simulink model "Torque_regulation_1_1"  (R2022b)
settings: Solver=FixedStepAuto  StartTime=0.0  StopTime=10  FixedStep=0.01  RelTol=1e-3
libraries: simulink x6, dspstat3 x4, eeGeneralControl x4, slpidlib x2
settings Model: Creator=tiszu  LastModifiedBy=tiszu

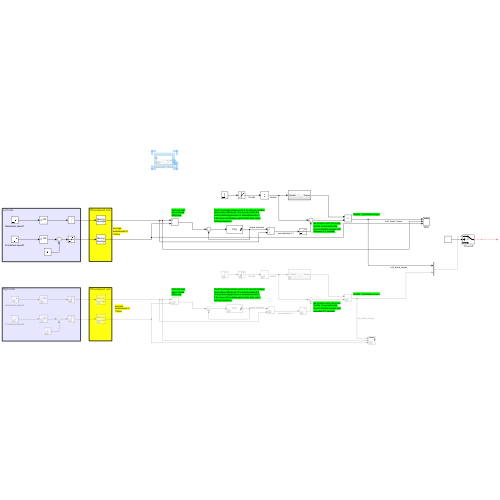
[thumbnail: Simulink's stored preview of the top-level diagram]
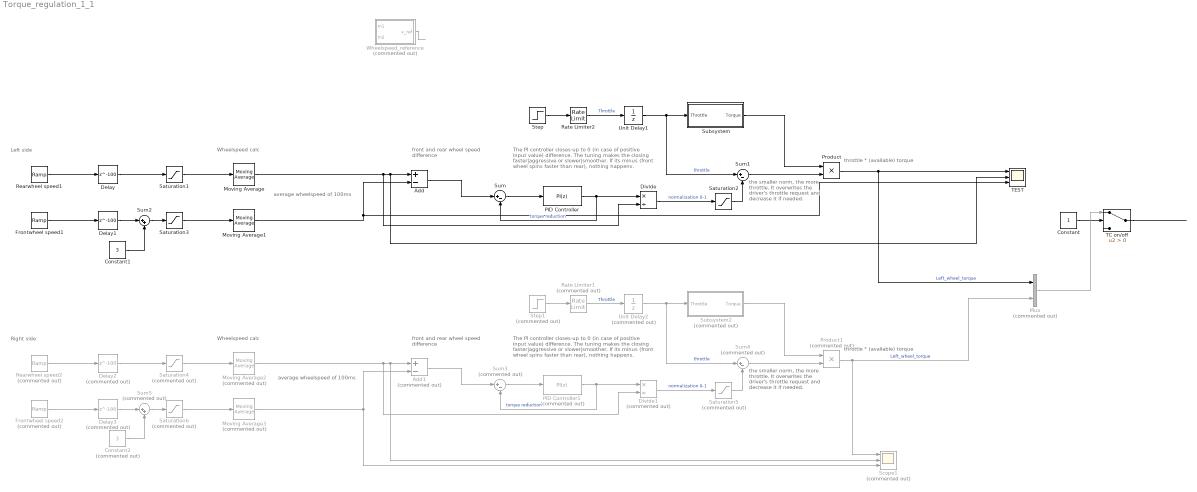
== system Torque_regulation_1_1 ==
  note: throttle * (available) torque
  note: the smaller norm, the more throttle. It overwrites the driver's throttle request and decrease it if needed.
  note: The PI controller closes-up to 0 (in case of positive input value) difference. The tuning makes the closing faster|aggressive or slower|smoother.
      | If its minus (front wheel spins faster than rear), nothing happens.
  note: average wheelspeed of 100ms
  note: Wheelspeed calc
  note: front and rear wheel speed difference
  note: Left side
  note: the smaller norm, the more throttle. It overwrites the driver's throttle request and decrease it if needed.
  note: Right side
  note: average wheelspeed of 100ms
  note: throttle * (available) torque
  note: The PI controller closes-up to 0 (in case of positive input value) difference. The tuning makes the closing faster|aggressive or slower|smoother.
      | If its minus (front wheel spins faster than rear), nothing happens.
  note: Wheelspeed calc
  note: front and rear wheel speed difference
  Add : Sum  Inputs=+-
  Add1 : Sum  Commented=on  Inputs=+-
  Constant : Constant
  Constant1 : Constant  Value=3
  Constant2 : Constant  Commented=on  Value=3
  Delay : Delay  DelayLength=100
  Delay1 : Delay  DelayLength=100
  Delay2 : Delay  Commented=on  DelayLength=100
  Delay3 : Delay  Commented=on  DelayLength=100
  Divide : Product  Inputs=*/
  Divide1 : Product  Commented=on  Inputs=*/
  Frontwheel speed1 : simulink/Sources/Ramp  slope=10  start=0  InitialOutput=0
  Frontwheel speed2 : simulink/Sources/Ramp  Commented=on  slope=10  start=0  InitialOutput=0
  Moving Average : dspstat3/Moving Average  Method=Sliding window  ForgettingFactorPort=off  SpecifyWindowLength=on  WindowLength=100  OverlapLength=99  AllowArbitraryInputLength=off  ForgettingFactor=0.9  SimulateUsing=Code generation
  Moving Average1 : dspstat3/Moving Average  Method=Sliding window  ForgettingFactorPort=off  SpecifyWindowLength=on  WindowLength=100  OverlapLength=99  AllowArbitraryInputLength=off  ForgettingFactor=0.9  SimulateUsing=Code generation
  Moving Average2 : dspstat3/Moving Average  Commented=on  Method=Sliding window  ForgettingFactorPort=off  SpecifyWindowLength=on  WindowLength=100  OverlapLength=99  AllowArbitraryInputLength=off  ForgettingFactor=0.9  SimulateUsing=Code generation
  Moving Average3 : dspstat3/Moving Average  Commented=on  Method=Sliding window  ForgettingFactorPort=off  SpecifyWindowLength=on  WindowLength=100  OverlapLength=99  AllowArbitraryInputLength=off  ForgettingFactor=0.9  SimulateUsing=Code generation
  Mux : Mux  Commented=on  Inputs=2
  PID Controller : slpidlib/PID Controller  Controller=PI  Form=Parallel  TimeDomain=Discrete-time  UseExternalTs=off  SampleTime=0.01  IntegratorMethod=Forward Euler  FilterMethod=Forward Euler  ControllerParametersSource=internal  P=1  I=2  UseKiTs=off  D=0  N=100  UseFilter=on  TunerSelectOption=Transfer Function Based (PID Tuner App)  InitialConditionSource=internal  InitialConditionForIntegrator=0  InitialConditionForFilter=0  DifferentiatorICPrevScaledInput=0  ExternalReset=none  TrackingMode=off  Kt=1  LimitOutput=on  SatLimitsSource=internal  UpperSaturationLimit=100  LowerSaturationLimit=0  LinearizeAsGain=on  AntiWindupMode=clamping  Kb=1  LimitIntegrator=off  UpperIntegratorSaturationLimit=inf  LowerIntegratorSaturationLimit=-inf  POutMin=[]  POutMax=[]  IOutMin=[]  IOutMax=[]  DOutMin=[]  DOutMax=[]  NOutMin=[]  NOutMax=[]  SumOutMin=[]  SumOutMax=[]  SaturationOutMin=[]  SaturationOutMax=[]  PParamMin=[]  PParamMax=[]  IParamMin=[]  IParamMax=[]  DParamMin=[]  DParamMax=[]  NParamMin=[]  NParamMax=[]  KbParamMin=[]  KbParamMax=[]  KtParamMin=[]  KtParamMax=[]  KbOutMin=[]  KbOutMax=[]  KtOutMin=[]  KtOutMax=[]  IntegratorOutMin=[]  IntegratorOutMax=[]  FilterOutMin=[]  FilterOutMax=[]  SumI1OutMin=[]  SumI1OutMax=[]  SumI2OutMin=[]  SumI2OutMax=[]  SumI3OutMin=[]  SumI3OutMax=[]  SumI4OutMin=[]  SumI4OutMax=[]  SumDOutMin=[]  SumDOutMax=[]  DifferentiatorOutMin=[]  DifferentiatorOutMax=[]  FilterDiffOutCoefMin=[]  FilterDiffOutCoefMax=[]  ReciprocalOutMin=[]  ReciprocalOutMax=[]  SumDenOutMin=[]  SumDenOutMax=[]  SumNumOutMin=[]  SumNumOutMax=[]  DivideOutMin=[]  DivideOutMax=[]  UdiffTsProdOutMin=[]  UdiffTsProdOutMax=[]  NTsProdOutMin=[]  NTsProdOutMax=[]  UintegralTsProdOutMin=[]  UintegralTsProdOutMax=[]  UngainTsProdOutMin=[]  UngainTsProdOutMax=[]  ClampingZeroOutDataTypeStr=Inherit: Inherit via back propagation  ClampingZeroOutMin=[]  ClampingZeroOutMax=[]  FilterDenConstantOutDataTypeStr=Inherit: Inherit via back propagation  FilterDenConstantOutMin=[]  FilterDenConstantOutMax=[]  PCopyOutDataTypeStr=Inherit: Inherit via back propagation  PCopyOutMin=[]  PCopyOutMax=[]  NCopyOutDataTypeStr=Inherit: Inherit via back propagation  NCopyOutMin=[]  NCopyOutMax=[]  IntegratorContinuousStateAttributes=''  IntegratorStateMustResolveToSignalObject=off  IntegratorRTWStateStorageClass=Auto  FilterContinuousStateAttributes=''  FilterStateMustResolveToSignalObject=off  FilterRTWStateStorageClass=Auto  ParallelPVariant=InternalParameters  IdealPVariant=Disabled  IVariant=InternalParameters  DVariant=Disabled  IntegratorVariant=Discrete  SatVariant=Enabled  AWVariant=DiscClampingParallel  PCopyVariant=Disabled  TRVariant=Disabled  FdbkBlocksVariant=Forward  IdealPFdbkVariant=Disabled  SatFdbkVariant=Disabled  DerivativeFilterVariant=Disabled  NVariant=Disabled  NCopyVariant=Disabled_SignalSpec  FilterICVariant=Disabled  IntegratorICVariant=InternalICs  ExternalResetVariant=Disabled  TRSumVariant=Passthrough  SumFdbkVariant=Disabled  SumVariant=Sum_PI  TsampFilterVariant=InternalTs  TsampNgainVariant=Passthrough  TsampIntegralVariant=Passthrough  ExternalSaturationOutDataTypeStr=Inherit: Same as second input
  PID Controller1 : slpidlib/PID Controller  Commented=on  Controller=PI  Form=Parallel  TimeDomain=Discrete-time  UseExternalTs=off  SampleTime=0.01  IntegratorMethod=Forward Euler  FilterMethod=Forward Euler  ControllerParametersSource=internal  P=1  I=2  UseKiTs=off  D=0  N=100  UseFilter=on  TunerSelectOption=Transfer Function Based (PID Tuner App)  InitialConditionSource=internal  InitialConditionForIntegrator=0  InitialConditionForFilter=0  DifferentiatorICPrevScaledInput=0  ExternalReset=none  TrackingMode=off  Kt=1  LimitOutput=on  SatLimitsSource=internal  UpperSaturationLimit=100  LowerSaturationLimit=0  LinearizeAsGain=on  AntiWindupMode=clamping  Kb=1  LimitIntegrator=off  UpperIntegratorSaturationLimit=inf  LowerIntegratorSaturationLimit=-inf  POutMin=[]  POutMax=[]  IOutMin=[]  IOutMax=[]  DOutMin=[]  DOutMax=[]  NOutMin=[]  NOutMax=[]  SumOutMin=[]  SumOutMax=[]  SaturationOutMin=[]  SaturationOutMax=[]  PParamMin=[]  PParamMax=[]  IParamMin=[]  IParamMax=[]  DParamMin=[]  DParamMax=[]  NParamMin=[]  NParamMax=[]  KbParamMin=[]  KbParamMax=[]  KtParamMin=[]  KtParamMax=[]  KbOutMin=[]  KbOutMax=[]  KtOutMin=[]  KtOutMax=[]  IntegratorOutMin=[]  IntegratorOutMax=[]  FilterOutMin=[]  FilterOutMax=[]  SumI1OutMin=[]  SumI1OutMax=[]  SumI2OutMin=[]  SumI2OutMax=[]  SumI3OutMin=[]  SumI3OutMax=[]  SumI4OutMin=[]  SumI4OutMax=[]  SumDOutMin=[]  SumDOutMax=[]  DifferentiatorOutMin=[]  DifferentiatorOutMax=[]  FilterDiffOutCoefMin=[]  FilterDiffOutCoefMax=[]  ReciprocalOutMin=[]  ReciprocalOutMax=[]  SumDenOutMin=[]  SumDenOutMax=[]  SumNumOutMin=[]  SumNumOutMax=[]  DivideOutMin=[]  DivideOutMax=[]  UdiffTsProdOutMin=[]  UdiffTsProdOutMax=[]  NTsProdOutMin=[]  NTsProdOutMax=[]  UintegralTsProdOutMin=[]  UintegralTsProdOutMax=[]  UngainTsProdOutMin=[]  UngainTsProdOutMax=[]  ClampingZeroOutDataTypeStr=Inherit: Inherit via back propagation  ClampingZeroOutMin=[]  ClampingZeroOutMax=[]  FilterDenConstantOutDataTypeStr=Inherit: Inherit via back propagation  FilterDenConstantOutMin=[]  FilterDenConstantOutMax=[]  PCopyOutDataTypeStr=Inherit: Inherit via back propagation  PCopyOutMin=[]  PCopyOutMax=[]  NCopyOutDataTypeStr=Inherit: Inherit via back propagation  NCopyOutMin=[]  NCopyOutMax=[]  IntegratorContinuousStateAttributes=''  IntegratorStateMustResolveToSignalObject=off  IntegratorRTWStateStorageClass=Auto  FilterContinuousStateAttributes=''  FilterStateMustResolveToSignalObject=off  FilterRTWStateStorageClass=Auto  ParallelPVariant=InternalParameters  IdealPVariant=Disabled  IVariant=InternalParameters  DVariant=Disabled  IntegratorVariant=Discrete  SatVariant=Enabled  AWVariant=DiscClampingParallel  PCopyVariant=Disabled  TRVariant=Disabled  FdbkBlocksVariant=Forward  IdealPFdbkVariant=Disabled  SatFdbkVariant=Disabled  DerivativeFilterVariant=Disabled  NVariant=Disabled  NCopyVariant=Disabled_SignalSpec  FilterICVariant=Disabled  IntegratorICVariant=InternalICs  ExternalResetVariant=Disabled  TRSumVariant=Passthrough  SumFdbkVariant=Disabled  SumVariant=Sum_PI  TsampFilterVariant=InternalTs  TsampNgainVariant=Passthrough  TsampIntegralVariant=Passthrough  ExternalSaturationOutDataTypeStr=Inherit: Same as second input
  Product : Product
  Product1 : Product  Commented=on
  Rate Limiter1 : RateLimiter  Commented=on  SampleTimeMode=inherited
  Rate Limiter2 : RateLimiter  SampleTimeMode=inherited
  Rearwheel speed1 : simulink/Sources/Ramp  slope=50  start=0  InitialOutput=0
  Rearwheel speed2 : simulink/Sources/Ramp  Commented=on  slope=50  start=0  InitialOutput=0
  Saturation1 : Saturate  UpperLimit=30  LowerLimit=0
  Saturation2 : Saturate  UpperLimit=1  LowerLimit=0
  Saturation3 : Saturate  UpperLimit=30  LowerLimit=0
  Saturation4 : Saturate  Commented=on  UpperLimit=30  LowerLimit=0
  Saturation5 : Saturate  Commented=on  UpperLimit=1  LowerLimit=0
  Saturation6 : Saturate  Commented=on  UpperLimit=30  LowerLimit=0
  Scope1 : Scope  Commented=on  NumInputPorts=3
  Step : Step  SampleTime=0
  Step1 : Step  Commented=on  SampleTime=0
  Subsystem : Subsystem
  Subsystem2 : Subsystem  Commented=on
  Sum : Sum  Inputs=|+-
  Sum1 : Sum  Inputs=|+-
  Sum2 : Sum  Inputs=|++
  Sum3 : Sum  Commented=on  Inputs=|+-
  Sum4 : Sum  Commented=on  Inputs=|+-
  Sum5 : Sum  Commented=on  Inputs=|++
  TC on/off : Switch  Criteria=u2 > Threshold  SaturateOnIntegerOverflow=off  InputSameDT=off
  TEST : Scope  NumInputPorts=3
  Unit Delay1 : UnitDelay  SampleTime=-1  HasFrameUpgradeWarning=on
  Unit Delay2 : UnitDelay  Commented=on  SampleTime=-1  HasFrameUpgradeWarning=on
  Wheelspeed_reference : Subsystem  Commented=on
  wires:
  Subsystem/1(Torque) -> Product/1
  Divide/1 -> Saturation2/1  "normalization 0-1"
  Sum1/1 -> Product/2
  PID Controller/1 -> Sum/2, Divide/1  "torque reduction"
  Saturation2/1 -> Sum1/2
  Wheelspeed_reference/1(v_ref) -> ?
  Sum2/1 -> Saturation3/1
  Sum/1 -> PID Controller/1
  Add/1 -> Sum/1
  Saturation1/1 -> Moving Average/1
  Saturation3/1 -> Moving Average1/1
  Delay/1 -> Saturation1/1
  Delay1/1 -> Sum2/1
  Rearwheel speed1/1 -> Delay/1
  Frontwheel speed1/1 -> Delay1/1
  Step/1 -> Rate Limiter2/1
  Rate Limiter2/1 -> Unit Delay1/1  "Throttle"
  Unit Delay1/1 -> Sum1/1, Subsystem/1(Throttle)  "throttle"
  Constant/1 -> TC on/off/2
  Mux/1 -> TC on/off/1
  TC on/off/1 -> ?
  Product/1 -> TEST/1, Mux/1  "Left_wheel_torque"
  Constant1/1 -> Sum2/2
  Moving Average/1 -> Divide/2, TEST/2, Add/1
  Moving Average1/1 -> Add/2, TEST/3
  Frontwheel speed2/1 -> Delay3/1
  Rate Limiter1/1 -> Unit Delay2/1  "Throttle"
  Subsystem2/1(Torque) -> Product1/1
  Sum4/1 -> Product1/2
  Unit Delay2/1 -> Sum4/1, Subsystem2/1(Throttle)  "throttle"
  Product1/1 -> Scope1/1, Mux/2  "Left_wheel_torque"
  Moving Average3/1 -> Add1/2, Scope1/3
  Constant2/1 -> Sum5/2
  Rearwheel speed2/1 -> Delay2/1
  Moving Average2/1 -> Divide1/2, Scope1/2, Add1/1
  Step1/1 -> Rate Limiter1/1
  Saturation6/1 -> Moving Average3/1
  Delay3/1 -> Sum5/1
  Delay2/1 -> Saturation4/1
  Saturation5/1 -> Sum4/2
  Sum3/1 -> PID Controller1/1
  Divide1/1 -> Saturation5/1  "normalization 0-1"
  Add1/1 -> Sum3/1
  Saturation4/1 -> Moving Average2/1
  Sum5/1 -> Saturation6/1
  PID Controller1/1 -> Sum3/2, Divide1/1  "torque reduction"

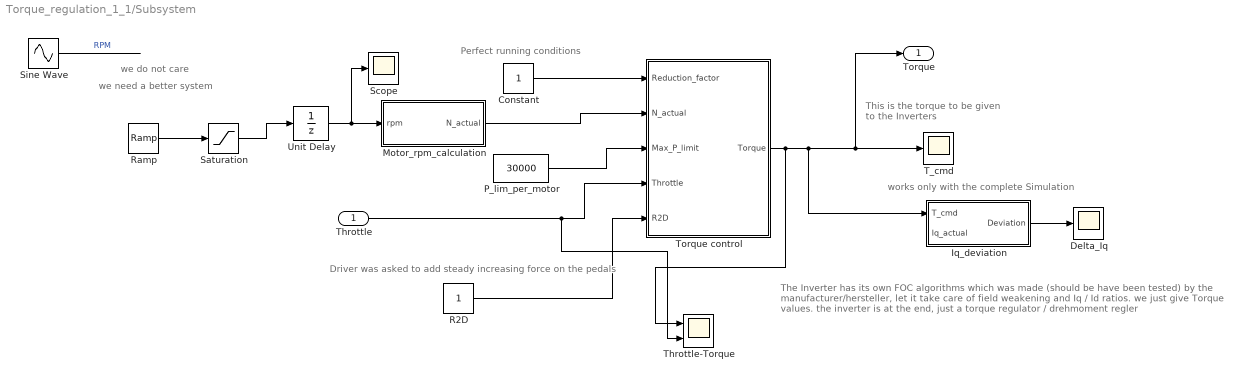
== system Torque_regulation_1_1/Subsystem ==
  note: we need a better system
  note: works only with the complete Simulation
  note: Perfect running conditions
  note: we do not care
  note: Driver was asked to add steady increasing force on the pedals
  note: The Inverter has its own FOC algorithms which was made (should be have been tested) by the manufacturer/hersteller, let it take care of field weakening and Iq / Id ratios. we just give Torque values. the inverter is at the end, just a torque regulator / drehmoment regler
  note: This is the torque to
      | be given to the Inverters
  Throttle : Inport
  Constant : Constant
  Delta_Iq : Scope
  Iq_deviation : Subsystem
  Motor_rpm_calculation : Subsystem
  P_lim_per_motor : Constant  Value=30000
  R2D : Constant
  Ramp : simulink/Sources/Ramp  slope=1000  start=0  InitialOutput=0
  Saturation : Saturate  UpperLimit=2000  LowerLimit=0
  Scope : Scope
  Sine Wave : Sin  Amplitude=2000  SampleTime=0
  T_cmd : Scope
  Throttle-Torque : Scope  NumInputPorts=2
  Torque control : Subsystem
  Unit Delay : UnitDelay  SampleTime=-1  HasFrameUpgradeWarning=on
  Torque : Outport
  wires:
  Throttle/1 -> Throttle-Torque/2, Torque control/4(Throttle)
  R2D/1 -> Torque control/5(R2D)
  Torque control/1(Torque) -> Iq_deviation/1(T_cmd), Torque/1, T_cmd/1, Throttle-Torque/1
  Unit Delay/1 -> Scope/1, Motor_rpm_calculation/1(rpm)
  Iq_deviation/1(Deviation) -> Delta_Iq/1
  Motor_rpm_calculation/1(N_actual) -> Torque control/2(N_actual)
  Sine Wave/1 -> ?  "RPM"
  Ramp/1 -> Saturation/1
  P_lim_per_motor/1 -> Torque control/3(Max_P_limit)
  Saturation/1 -> Unit Delay/1
  Constant/1 -> Torque control/1(Reduction_factor)

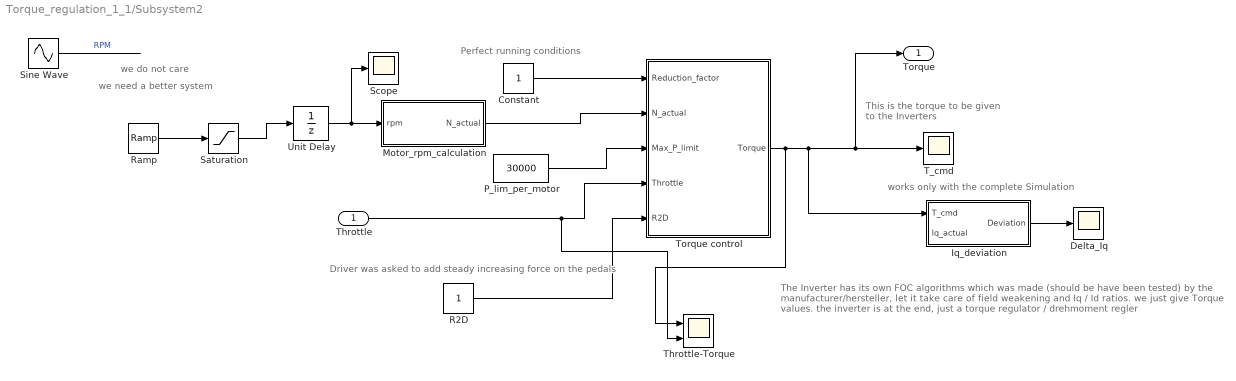
== system Torque_regulation_1_1/Subsystem2 ==
  note: we need a better system
  note: works only with the complete Simulation
  note: Perfect running conditions
  note: we do not care
  note: Driver was asked to add steady increasing force on the pedals
  note: The Inverter has its own FOC algorithms which was made (should be have been tested) by the manufacturer/hersteller, let it take care of field weakening and Iq / Id ratios. we just give Torque values. the inverter is at the end, just a torque regulator / drehmoment regler
  note: This is the torque to
      | be given to the Inverters
  Throttle : Inport
  Constant : Constant
  Delta_Iq : Scope
  Iq_deviation : Subsystem
  Motor_rpm_calculation : Subsystem
  P_lim_per_motor : Constant  Value=30000
  R2D : Constant
  Ramp : simulink/Sources/Ramp  slope=1000  start=0  InitialOutput=0
  Saturation : Saturate  UpperLimit=2000  LowerLimit=0
  Scope : Scope
  Sine Wave : Sin  Amplitude=2000  SampleTime=0
  T_cmd : Scope
  Throttle-Torque : Scope  NumInputPorts=2
  Torque control : Subsystem
  Unit Delay : UnitDelay  SampleTime=-1  HasFrameUpgradeWarning=on
  Torque : Outport
  wires:
  Throttle/1 -> Throttle-Torque/2, Torque control/4(Throttle)
  R2D/1 -> Torque control/5(R2D)
  Torque control/1(Torque) -> Iq_deviation/1(T_cmd), Torque/1, T_cmd/1, Throttle-Torque/1
  Unit Delay/1 -> Scope/1, Motor_rpm_calculation/1(rpm)
  Iq_deviation/1(Deviation) -> Delta_Iq/1
  Motor_rpm_calculation/1(N_actual) -> Torque control/2(N_actual)
  Sine Wave/1 -> ?  "RPM"
  Ramp/1 -> Saturation/1
  P_lim_per_motor/1 -> Torque control/3(Max_P_limit)
  Saturation/1 -> Unit Delay/1
  Constant/1 -> Torque control/1(Reduction_factor)

== system Torque_regulation_1_1/Wheelspeed_reference ==
  In1 : Inport
  In2 : Inport  Port=2
  Min : MinMax  Inputs=2
  v_ref : Outport
  wires:
  In1/1 -> Min/1
  Min/1 -> v_ref/1
  In2/1 -> Min/2

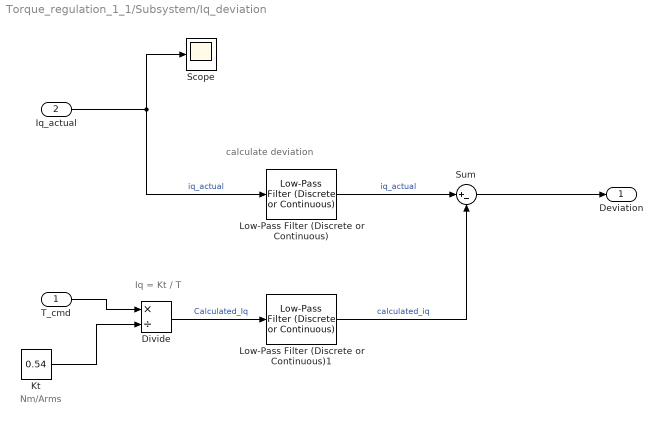
== system Torque_regulation_1_1/Subsystem/Iq_deviation ==
  note: calculate deviation
  note: Iq = Kt / T
  note: Nm/Arms
  T_cmd : Inport
  Iq_actual : Inport  Port=2
  Divide : Product  Inputs=*/
  Kt : Constant  Value=0.54
  Low-Pass Filter (Discrete or Continuous) : eeGeneralControl/Low-Pass Filter (Discrete or Continuous)  K=1  T=1  B=inf  A=-inf  init_option=Inherited from block input  x0=0  Ts=-1
  Low-Pass Filter (Discrete or Continuous)1 : eeGeneralControl/Low-Pass Filter (Discrete or Continuous)  K=1  T=1  B=inf  A=-inf  init_option=Inherited from block input  x0=0  Ts=-1
  Scope : Scope
  Sum : Sum  Inputs=|+-
  Deviation : Outport
  wires:
  Kt/1 -> Divide/2
  T_cmd/1 -> Divide/1
  Iq_actual/1 -> Low-Pass Filter (Discrete or Continuous)/1, Scope/1  "iq_actual"
  Divide/1 -> Low-Pass Filter (Discrete or Continuous)1/1  "Calculated_Iq"
  Sum/1 -> Deviation/1
  Low-Pass Filter (Discrete or Continuous)/1 -> Sum/1  "iq_actual"
  Low-Pass Filter (Discrete or Continuous)1/1 -> Sum/2  "calculated_iq"

== system Torque_regulation_1_1/Subsystem/Motor_rpm_calculation ==
  note: From CAN Docs Pg 19
      | (Unitek)
  rpm : Inport
  15-Bit_Max_value : Constant  Value=32767
  Constant : Constant  Value=8000
  Divide : Product  Inputs=*/
  Product : Product
  N_actual : Outport
  wires:
  rpm/1 -> Divide/1
  Divide/1 -> Product/1
  15-Bit_Max_value/1 -> Product/2
  Constant/1 -> Divide/2
  Product/1 -> N_actual/1

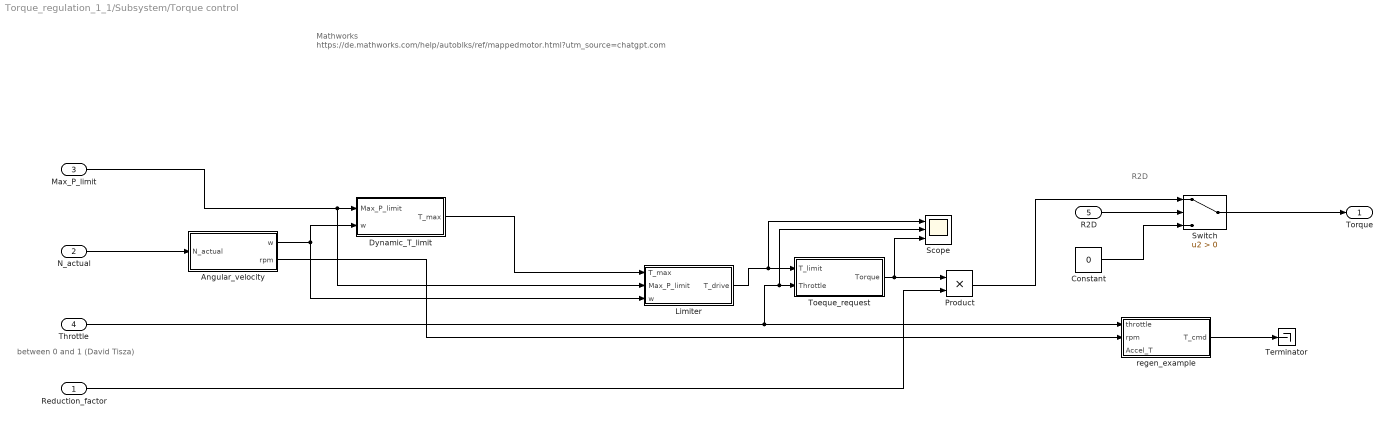
== system Torque_regulation_1_1/Subsystem/Torque control ==
  note: R2D
  note: between 0 and 1 (David Tisza)
  note: Mathworks
      | https://de.mathworks.com/help/autoblks/ref/mappedmotor.html?utm_source=chatgpt.com
  Reduction_factor : Inport
  N_actual : Inport  Port=2
  Max_P_limit : Inport  Port=3
  Throttle : Inport  Port=4
  R2D : Inport  Port=5
  Angular_velocity : Subsystem
  Constant : Constant  Value=0
  Dynamic_T_limit : Subsystem
  Limiter : Subsystem
  Product : Product
  Scope : Scope  NumInputPorts=3
  Switch : Switch  Criteria=u2 > Threshold  SaturateOnIntegerOverflow=off  InputSameDT=off
  Terminator : Terminator
  Toeque_request : Subsystem
  regen_example : Subsystem
  Torque : Outport
  wires:
  N_actual/1 -> Angular_velocity/1(N_actual)
  Throttle/1 -> regen_example/1(throttle), Scope/2, Toeque_request/2(Throttle)
  Angular_velocity/1(w) -> Limiter/3(w), Dynamic_T_limit/2(w)
  Max_P_limit/1 -> Limiter/2(Max_P_limit), Dynamic_T_limit/1(Max_P_limit)
  Limiter/1(T_drive) -> Scope/1, Toeque_request/1(T_limit)
  Toeque_request/1(Torque) -> Scope/3, Product/1
  Product/1 -> Switch/1
  Reduction_factor/1 -> Product/2
  Dynamic_T_limit/1(T_max) -> Limiter/1(T_max)
  Angular_velocity/2(rpm) -> regen_example/2(rpm)
  regen_example/1(T_cmd) -> Terminator/1
  R2D/1 -> Switch/2
  Constant/1 -> Switch/3
  Switch/1 -> Torque/1

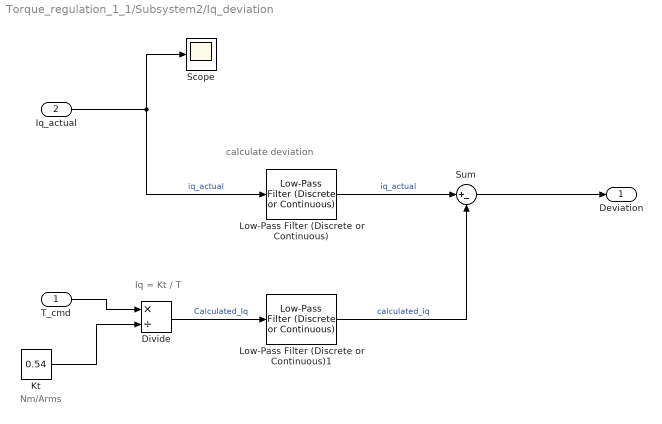
== system Torque_regulation_1_1/Subsystem2/Iq_deviation ==
  note: calculate deviation
  note: Iq = Kt / T
  note: Nm/Arms
  T_cmd : Inport
  Iq_actual : Inport  Port=2
  Divide : Product  Inputs=*/
  Kt : Constant  Value=0.54
  Low-Pass Filter (Discrete or Continuous) : eeGeneralControl/Low-Pass Filter (Discrete or Continuous)  K=1  T=1  B=inf  A=-inf  init_option=Inherited from block input  x0=0  Ts=-1
  Low-Pass Filter (Discrete or Continuous)1 : eeGeneralControl/Low-Pass Filter (Discrete or Continuous)  K=1  T=1  B=inf  A=-inf  init_option=Inherited from block input  x0=0  Ts=-1
  Scope : Scope
  Sum : Sum  Inputs=|+-
  Deviation : Outport
  wires:
  Kt/1 -> Divide/2
  T_cmd/1 -> Divide/1
  Iq_actual/1 -> Low-Pass Filter (Discrete or Continuous)/1, Scope/1  "iq_actual"
  Divide/1 -> Low-Pass Filter (Discrete or Continuous)1/1  "Calculated_Iq"
  Sum/1 -> Deviation/1
  Low-Pass Filter (Discrete or Continuous)/1 -> Sum/1  "iq_actual"
  Low-Pass Filter (Discrete or Continuous)1/1 -> Sum/2  "calculated_iq"

== system Torque_regulation_1_1/Subsystem2/Motor_rpm_calculation ==
  note: From CAN Docs Pg 19
      | (Unitek)
  rpm : Inport
  15-Bit_Max_value : Constant  Value=32767
  Constant : Constant  Value=8000
  Divide : Product  Inputs=*/
  Product : Product
  N_actual : Outport
  wires:
  rpm/1 -> Divide/1
  Divide/1 -> Product/1
  15-Bit_Max_value/1 -> Product/2
  Constant/1 -> Divide/2
  Product/1 -> N_actual/1

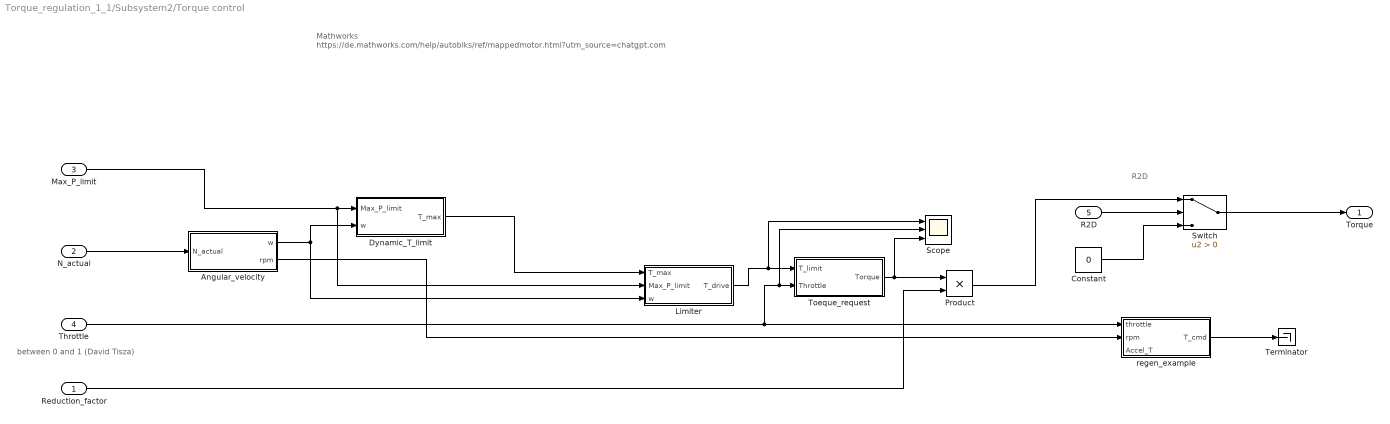
== system Torque_regulation_1_1/Subsystem2/Torque control ==
  note: R2D
  note: between 0 and 1 (David Tisza)
  note: Mathworks
      | https://de.mathworks.com/help/autoblks/ref/mappedmotor.html?utm_source=chatgpt.com
  Reduction_factor : Inport
  N_actual : Inport  Port=2
  Max_P_limit : Inport  Port=3
  Throttle : Inport  Port=4
  R2D : Inport  Port=5
  Angular_velocity : Subsystem
  Constant : Constant  Value=0
  Dynamic_T_limit : Subsystem
  Limiter : Subsystem
  Product : Product
  Scope : Scope  NumInputPorts=3
  Switch : Switch  Criteria=u2 > Threshold  SaturateOnIntegerOverflow=off  InputSameDT=off
  Terminator : Terminator
  Toeque_request : Subsystem
  regen_example : Subsystem
  Torque : Outport
  wires:
  N_actual/1 -> Angular_velocity/1(N_actual)
  Throttle/1 -> regen_example/1(throttle), Scope/2, Toeque_request/2(Throttle)
  Angular_velocity/1(w) -> Limiter/3(w), Dynamic_T_limit/2(w)
  Max_P_limit/1 -> Limiter/2(Max_P_limit), Dynamic_T_limit/1(Max_P_limit)
  Limiter/1(T_drive) -> Scope/1, Toeque_request/1(T_limit)
  Toeque_request/1(Torque) -> Scope/3, Product/1
  Product/1 -> Switch/1
  Reduction_factor/1 -> Product/2
  Dynamic_T_limit/1(T_max) -> Limiter/1(T_max)
  Angular_velocity/2(rpm) -> regen_example/2(rpm)
  regen_example/1(T_cmd) -> Terminator/1
  R2D/1 -> Switch/2
  Constant/1 -> Switch/3
  Switch/1 -> Torque/1

== system Torque_regulation_1_1/Subsystem/Torque control/Angular_velocity ==
  note: Angular velocity in
      | rad / s
  note: per Minute, therefore / 60
  note: value from Inverter (is not RPM)
  note: well lets say max rpm = 8000 (EMRAX 188 MAX)
  N_actual : Inport
  Constant : Constant  Value=8000
  Gain : Gain  Gain=(2*pi) / 60
  Motor_rpm_calculation : Subsystem
  Scope : Scope  NumInputPorts=2
  w : Outport
  rpm : Outport  Port=2
  wires:
  N_actual/1 -> Motor_rpm_calculation/2(N_actual)
  Constant/1 -> Motor_rpm_calculation/1(rpm_max)
  Gain/1 -> Scope/2, w/1  "rad/s"
  Motor_rpm_calculation/1(Motor_rpm) -> rpm/1, Scope/1, Gain/1

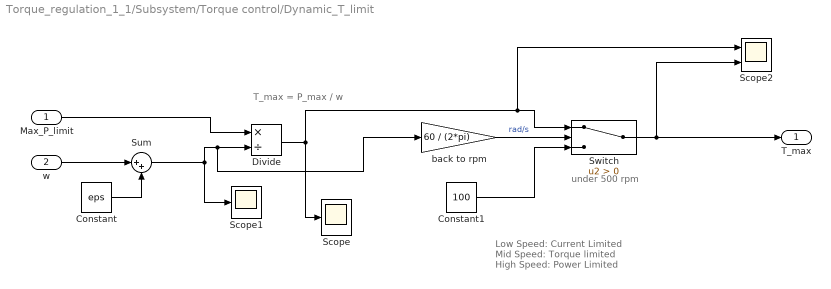
== system Torque_regulation_1_1/Subsystem/Torque control/Dynamic_T_limit ==
  note: under 500 rpm
  note: Low Speed: Current Limited
      | Mid Speed: Torque limited
      | High Speed: Power Limited
  note: T_max = P_max / w
  Max_P_limit : Inport
  w : Inport  Port=2
  Constant : Constant  Value=eps
  Constant1 : Constant  Value=100
  Divide : Product  Inputs=*/
  Scope : Scope
  Scope1 : Scope
  Scope2 : Scope  NumInputPorts=2
  Sum : Sum  Inputs=|++
  Switch : Switch  Criteria=u2 > Threshold  SaturateOnIntegerOverflow=off  InputSameDT=off
  "back to rpm " : Gain  Gain=60 / (2*pi)
  T_max : Outport
  wires:
  Sum/1 -> Scope1/1, "back to rpm "/1, Divide/2
  Max_P_limit/1 -> Divide/1
  Divide/1 -> Scope/1, Scope2/1, Switch/1
  Constant/1 -> Sum/2
  w/1 -> Sum/1
  Switch/1 -> Scope2/2, T_max/1
  "back to rpm "/1 -> Switch/2  "rad/s"
  Constant1/1 -> Switch/3

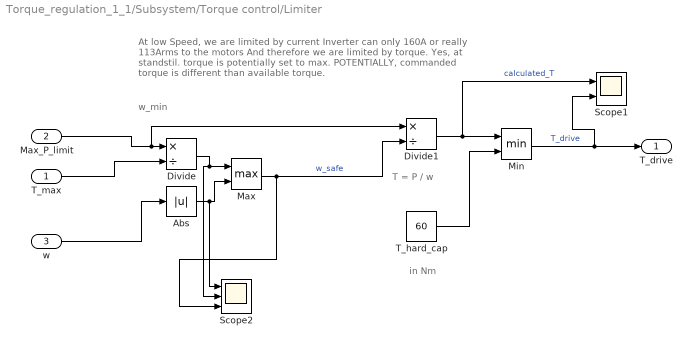
== system Torque_regulation_1_1/Subsystem/Torque control/Limiter ==
  note: T = P / w
  note: in Nm
  note: At low Speed, we are limited by current
      | Inverter can only 160A or really 113Arms to the motors
      |
      | And therefore we are limited by torque.
      | Yes, at standstil. torque is potentially set to max.
      | POTENTIALLY, commanded torque is different than available torque.
  note: w_min
  T_max : Inport
  Max_P_limit : Inport  Port=2
  w : Inport  Port=3
  Abs : Abs  SaturateOnIntegerOverflow=off
  Divide : Product  Inputs=*/
  Divide1 : Product  Inputs=*/
  Max : MinMax  Function=max  Inputs=2
  Min : MinMax  Inputs=2
  Scope1 : Scope  NumInputPorts=2
  Scope2 : Scope  NumInputPorts=3
  T_hard_cap : Constant  Value=60
  T_drive : Outport
  wires:
  Max_P_limit/1 -> Divide1/1, Divide/1
  T_max/1 -> Divide/2
  w/1 -> Abs/1
  Divide/1 -> Max/1, Scope2/2
  Abs/1 -> Scope2/1, Max/2
  Max/1 -> Divide1/2, Scope2/3  "w_safe"
  Divide1/1 -> Scope1/1, Min/1  "calculated_T"
  T_hard_cap/1 -> Min/2
  Min/1 -> Scope1/2, T_drive/1  "T_drive"

== system Torque_regulation_1_1/Subsystem/Torque control/Toeque_request ==
  note: T = u * T_max
  note: Between 1 and 0
  T_limit : Inport
  Throttle : Inport  Port=2
  Product : Product
  Saturation : Saturate  UpperLimit=1  LowerLimit=0
  Torque : Outport
  wires:
  Throttle/1 -> Saturation/1
  Saturation/1 -> Product/1
  T_limit/1 -> Product/2
  Product/1 -> Torque/1

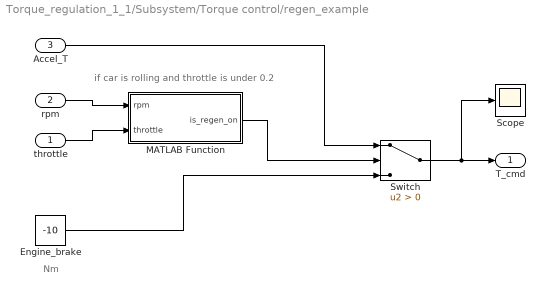
== system Torque_regulation_1_1/Subsystem/Torque control/regen_example ==
  note: if car is rolling and throttle is under 0.2
  note: Nm
  throttle : Inport
  rpm : Inport  Port=2
  Accel_T : Inport  Port=3
  Engine_brake : Constant  Value=-10
  MATLAB Function : MATLAB Function  TreatAsAtomicUnit=on
  Scope : Scope
  Switch : Switch  Criteria=u2 > Threshold  SaturateOnIntegerOverflow=off  InputSameDT=off
  T_cmd : Outport
  wires:
  Accel_T/1 -> Switch/1
  throttle/1 -> MATLAB Function/2(throttle)
  rpm/1 -> MATLAB Function/1(rpm)
  MATLAB Function/1(is_regen_on) -> Switch/2
  Engine_brake/1 -> Switch/3
  Switch/1 -> Scope/1, T_cmd/1

== system Torque_regulation_1_1/Subsystem2/Torque control/Angular_velocity ==
  note: Angular velocity in
      | rad / s
  note: per Minute, therefore / 60
  note: value from Inverter (is not RPM)
  note: well lets say max rpm = 8000 (EMRAX 188 MAX)
  N_actual : Inport
  Constant : Constant  Value=8000
  Gain : Gain  Gain=(2*pi) / 60
  Motor_rpm_calculation : Subsystem
  Scope : Scope  NumInputPorts=2
  w : Outport
  rpm : Outport  Port=2
  wires:
  N_actual/1 -> Motor_rpm_calculation/2(N_actual)
  Constant/1 -> Motor_rpm_calculation/1(rpm_max)
  Gain/1 -> Scope/2, w/1  "rad/s"
  Motor_rpm_calculation/1(Motor_rpm) -> rpm/1, Scope/1, Gain/1

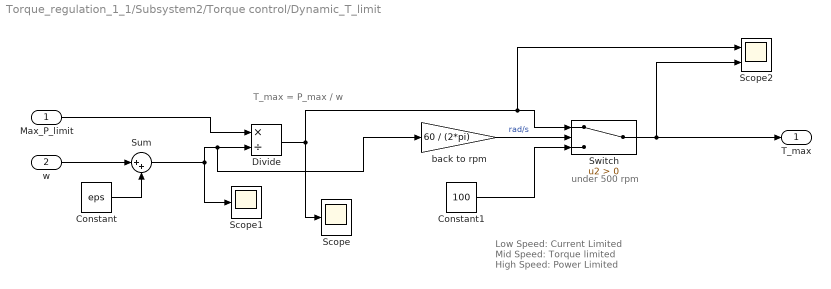
== system Torque_regulation_1_1/Subsystem2/Torque control/Dynamic_T_limit ==
  note: under 500 rpm
  note: Low Speed: Current Limited
      | Mid Speed: Torque limited
      | High Speed: Power Limited
  note: T_max = P_max / w
  Max_P_limit : Inport
  w : Inport  Port=2
  Constant : Constant  Value=eps
  Constant1 : Constant  Value=100
  Divide : Product  Inputs=*/
  Scope : Scope
  Scope1 : Scope
  Scope2 : Scope  NumInputPorts=2
  Sum : Sum  Inputs=|++
  Switch : Switch  Criteria=u2 > Threshold  SaturateOnIntegerOverflow=off  InputSameDT=off
  "back to rpm " : Gain  Gain=60 / (2*pi)
  T_max : Outport
  wires:
  Sum/1 -> Scope1/1, "back to rpm "/1, Divide/2
  Max_P_limit/1 -> Divide/1
  Divide/1 -> Scope/1, Scope2/1, Switch/1
  Constant/1 -> Sum/2
  w/1 -> Sum/1
  Switch/1 -> Scope2/2, T_max/1
  "back to rpm "/1 -> Switch/2  "rad/s"
  Constant1/1 -> Switch/3

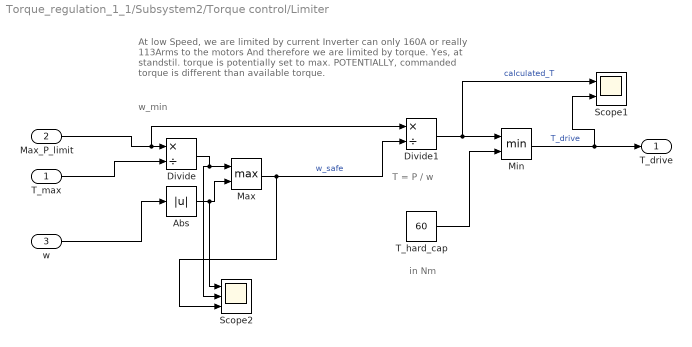
== system Torque_regulation_1_1/Subsystem2/Torque control/Limiter ==
  note: T = P / w
  note: in Nm
  note: At low Speed, we are limited by current
      | Inverter can only 160A or really 113Arms to the motors
      |
      | And therefore we are limited by torque.
      | Yes, at standstil. torque is potentially set to max.
      | POTENTIALLY, commanded torque is different than available torque.
  note: w_min
  T_max : Inport
  Max_P_limit : Inport  Port=2
  w : Inport  Port=3
  Abs : Abs  SaturateOnIntegerOverflow=off
  Divide : Product  Inputs=*/
  Divide1 : Product  Inputs=*/
  Max : MinMax  Function=max  Inputs=2
  Min : MinMax  Inputs=2
  Scope1 : Scope  NumInputPorts=2
  Scope2 : Scope  NumInputPorts=3
  T_hard_cap : Constant  Value=60
  T_drive : Outport
  wires:
  Max_P_limit/1 -> Divide1/1, Divide/1
  T_max/1 -> Divide/2
  w/1 -> Abs/1
  Divide/1 -> Max/1, Scope2/2
  Abs/1 -> Scope2/1, Max/2
  Max/1 -> Divide1/2, Scope2/3  "w_safe"
  Divide1/1 -> Scope1/1, Min/1  "calculated_T"
  T_hard_cap/1 -> Min/2
  Min/1 -> Scope1/2, T_drive/1  "T_drive"

== system Torque_regulation_1_1/Subsystem2/Torque control/Toeque_request ==
  note: T = u * T_max
  note: Between 1 and 0
  T_limit : Inport
  Throttle : Inport  Port=2
  Product : Product
  Saturation : Saturate  UpperLimit=1  LowerLimit=0
  Torque : Outport
  wires:
  Throttle/1 -> Saturation/1
  Saturation/1 -> Product/1
  T_limit/1 -> Product/2
  Product/1 -> Torque/1

== system Torque_regulation_1_1/Subsystem2/Torque control/regen_example ==
  note: if car is rolling and throttle is under 0.2
  note: Nm
  throttle : Inport
  rpm : Inport  Port=2
  Accel_T : Inport  Port=3
  Engine_brake : Constant  Value=-10
  MATLAB Function : MATLAB Function  TreatAsAtomicUnit=on
  Scope : Scope
  Switch : Switch  Criteria=u2 > Threshold  SaturateOnIntegerOverflow=off  InputSameDT=off
  T_cmd : Outport
  wires:
  Accel_T/1 -> Switch/1
  throttle/1 -> MATLAB Function/2(throttle)
  rpm/1 -> MATLAB Function/1(rpm)
  MATLAB Function/1(is_regen_on) -> Switch/2
  Engine_brake/1 -> Switch/3
  Switch/1 -> Scope/1, T_cmd/1

== system Torque_regulation_1_1/Subsystem/Torque control/Angular_velocity/Motor_rpm_calculation ==
  note: From CAN Docs Pg 19
      | (Unitek)
  rpm_max : Inport
  N_actual : Inport  Port=2
  15-Bit_Max_value : Constant  Value=32767
  Divide : Product  Inputs=*/
  Product : Product
  Motor_rpm : Outport
  wires:
  N_actual/1 -> Divide/1
  Divide/1 -> Product/1
  15-Bit_Max_value/1 -> Divide/2
  rpm_max/1 -> Product/2
  Product/1 -> Motor_rpm/1

== system Torque_regulation_1_1/Subsystem2/Torque control/Angular_velocity/Motor_rpm_calculation ==
  note: From CAN Docs Pg 19
      | (Unitek)
  rpm_max : Inport
  N_actual : Inport  Port=2
  15-Bit_Max_value : Constant  Value=32767
  Divide : Product  Inputs=*/
  Product : Product
  Motor_rpm : Outport
  wires:
  N_actual/1 -> Divide/1
  Divide/1 -> Product/1
  15-Bit_Max_value/1 -> Divide/2
  rpm_max/1 -> Product/2
  Product/1 -> Motor_rpm/1

== matlab function Torque_regulation_1_1/Subsystem/Torque control/regen_example/MATLAB Function ==
  data: rpm input; is_regen_on output; throttle input
function is_regen_on = fcn(rpm, throttle)

if (rpm > 0 && throttle < 0.2)
    is_regen_on = 1;
else
    is_regen_on = 0;
end

== matlab function Torque_regulation_1_1/Subsystem2/Torque control/regen_example/MATLAB Function ==
  data: rpm input; is_regen_on output; throttle input
function is_regen_on = fcn(rpm, throttle)

if (rpm > 0 && throttle < 0.2)
    is_regen_on = 1;
else
    is_regen_on = 0;
end
